simulink model "Signal5"  (Simulink 8.3)
settings: Solver=ode45  StartTime=0.0  StopTime=20  RelTol=1e-3
settings Model: Creator=Admin  LastModifiedBy=stud507ikt
settings OptimizationCC: ExpressionDepthLimit=2147483647
settings DebuggingCC: FcnCallInpInsideContextMsg=EnableAllAsWarning
settings GRTTargetCC: CombineOutputUpdateFcns=on  GRTInterface=off

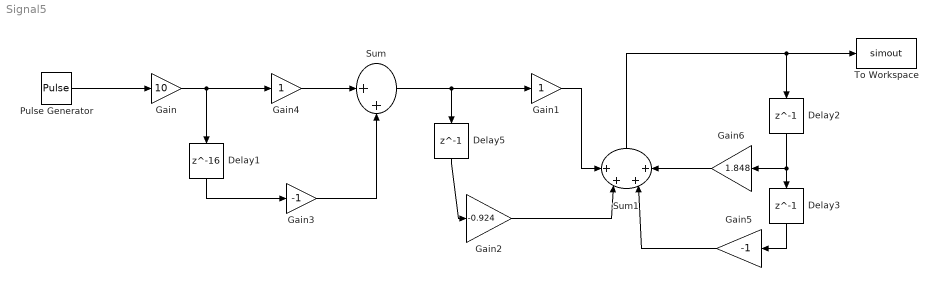
== system Signal5 ==
  Delay1 : Delay  DelayLength=16
  Delay2 : Delay  DelayLength=1
  Delay3 : Delay  DelayLength=1
  Delay5 : Delay  DelayLength=1
  Gain : Gain  Gain=10
  Gain1 : Gain
  Gain2 : Gain  Gain=-0.924
  Gain3 : Gain  Gain=-1
  Gain4 : Gain
  Gain5 : Gain  Gain=-1
  Gain6 : Gain  Gain=1.848
  Pulse Generator : DiscretePulseGenerator  Period=100
  Sum : Sum  Inputs=|++
  Sum1 : Sum  Inputs=++++
  To Workspace : ToWorkspace  VariableName=simout  SampleTime=-1
  wires:
  Pulse Generator/1 -> Gain/1
  Gain/1 -> Gain4/1, Delay1/1
  Gain4/1 -> Sum/1
  Sum/1 -> Gain1/1, Delay5/1
  Delay1/1 -> Gain3/1
  Gain3/1 -> Sum/2
  Delay5/1 -> Gain2/1
  Gain2/1 -> Sum1/2
  Gain1/1 -> Sum1/1
  Gain5/1 -> Sum1/3
  Gain6/1 -> Sum1/4
  Delay2/1 -> Delay3/1, Gain6/1
  Delay3/1 -> Gain5/1
  Sum1/1 -> To Workspace/1, Delay2/1
